simulink model "Lab2"  (R2017b)
settings: Solver=VariableStepAuto  StartTime=0.0  StopTime=10.0  RelTol=1e-3
settings Model: Creator=ArsalanBangash  LastModifiedBy=ArsalanBangash

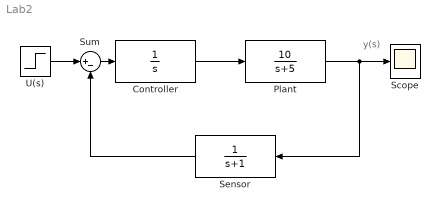
== system Lab2 ==
  note: y(s)
  Controller : TransferFcn  Denominator=[1 0]
  Plant : TransferFcn  Numerator=[10]  Denominator=[1 5]
  Scope : Scope
  Sensor : TransferFcn  Denominator=[1 1]
  Sum : Sum  Inputs=|+-
  U(s) : Step  SampleTime=0
  wires:
  Sum/1 -> Controller/1
  Controller/1 -> Plant/1
  Plant/1 -> Scope/1, Sensor/1
  Sensor/1 -> Sum/2
  U(s)/1 -> Sum/1
